simulink model "x2dof_manipulator_sim"  (R2025b)
settings: Solver=ode23t  StartTime=0.0  StopTime=simtime  RelTol=1e-3
values from neighbouring files (symbols this model uses):
  Kd = 3    [manip_parameters.m]
  Kp = 10    [manip_parameters.m]
  l1 = 0.6658    [manip_parameters.m]    (also in simscape_fitness.m = x(1))
  l2 = 0.3342    [manip_parameters.m]    (also in simscape_fitness.m = x(2))
  M = 5    [manip_parameters.m]
  R1 = 0.0102    [manip_parameters.m]    (also in simscape_fitness.m = x(3))
  R2 = 0.0101    [manip_parameters.m]    (also in simscape_fitness.m = x(4))
  thickness = 2/1000    (= 0.002)    [manip_parameters.m]
  X0 = l1    (= 0.6658)    [manip_parameters.m]
  Xf = 0.1    [manip_parameters.m]
  Z0 = (l1^2+l2^2)^(1/2)    (= 0.744969314804)    [manip_parameters.m]
  Zf = 0.5    [manip_parameters.m]
undefined symbols (not defined in the file or in its folder): X, Y, Z
libraries: sm_lib x12, nesl_utility x10
settings Model: Creator=david  LastModifiedBy=david
settings ExplorerConfigSet: InternalSimMechanicsExplorerSettings=|
  | <ExplorerConfiguration>
  | 
  |   <canonicalview>default</canonicalview>
  | 
  |   <TilePanel>
  |     <TileInfo>
  |       <Tiles Columns="1" Count="1" Height="608" Rows="1" Width="1079">
  |         <Row Weight="1"/>
  |         <Column Weight="1"/>
  |         <Tile Height="1" Width="1" X="0" Y="0"/>
  |       </Tiles>
  |     </TileInfo>
  |     <SceneInfo>
  |       <SceneViewer>
  |         <IsThisViewStd>
  |           <IsStandardView>off</IsStandardView>
  |           <StandardViewName>Front</StandardViewName>
  |         </IsThisViewStd>
  |         <BGColor>
  |           <R>1</R>
  |           <G>1</G>
  |           <B>1</B>
  |           <A>1</A>
  |         </BGColor>
  |         <Camera>
  |           <DoPerspective>off</DoPerspective>
  |           <Position>
  |             <X>0.46670638678844834</X>
  |             <Y>-2.3711199999999999</Y>
  |             <Z>0.2607597590218651</Z>
  |           </Position>
  |           <Center>
  |             <X>0.46670638678844834</X>
  |             <Y>0</Y>
  |             <Z>0.2607597590218651</Z>
  |           </Center>
  |           <Up>
  |             <X>0</X>
  |             <Y>0</Y>
  |             <Z>1</Z>
  |           </Up>
  |           <XLim>0.53368918601454662</XLim>
  |           <YLim>0.53368918601454662</YLim>
  |           <ViewLimDist>0.01</ViewLimDist>
  |         </Camera>
  |       </SceneViewer>
  |     </SceneInfo>
  |   </TilePanel>
  | 
  |   <MechEditorPanel>
  |     <GfxPanelCameraMap/>
  |     <Cameras/>
  |     <VideoCreator>
  |       <IncludeTiles>All</IncludeTiles>
  |       <IncludeTime>on</IncludeTime>
  |       <IncludeWorldFrame>off</IncludeWorldFrame>
  |       <PlaybackSpeedRatio>1</PlaybackSpeedRatio>
  |       <FrameRate>30</FrameRate>
  |       <FrameSize>auto</FrameSize>
  |       <VideoFormat>UncompressedAVI</VideoFormat>
  |     </VideoCreator>
  |   </MechEditorPanel>
  | 
  |   <PlaybackSettings>
  |     <PlaybackSpeedFactor>1</PlaybackSpeedFactor>
  |   </PlaybackSettings>
  | 
  | </ExplorerConfiguration>

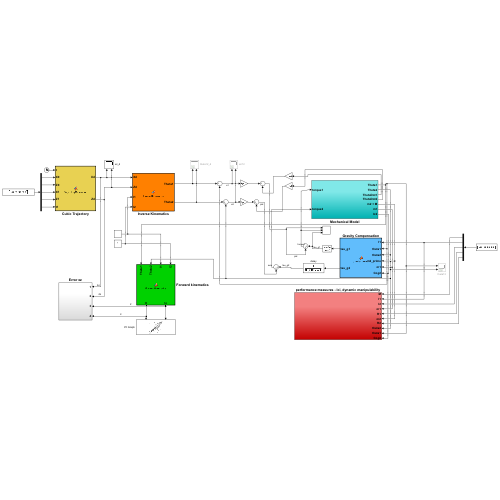
[thumbnail: Simulink's stored preview of the top-level diagram]
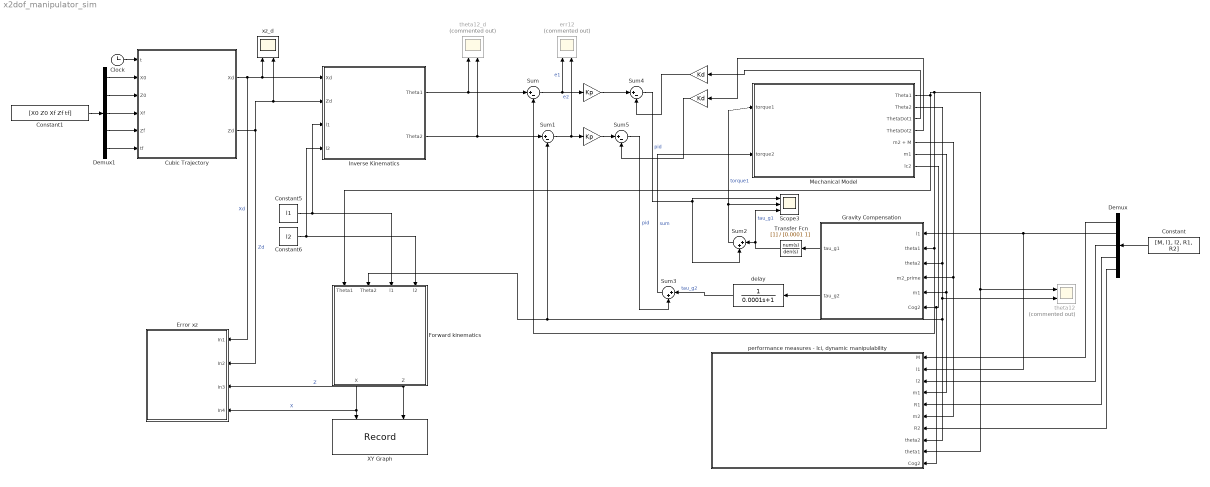
== system x2dof_manipulator_sim ==
  " " : Gain  Gain=Kd
  "  " : Gain  Gain=Kd
  "    " : Gain  Gain=Kp
  "     " : Gain  Gain=Kp
  Clock : Clock
  Constant : Constant  Value=[M, l1, l2, R1, R2]
  Constant1 : Constant  Value=[X0 Z0 Xf Zf tf]
  Constant5 : Constant  Value=l1
  Constant6 : Constant  Value=l2
  Cubic Trajectory : MATLAB Function  TreatAsAtomicUnit=on
  Demux : Demux  Outputs=5
  Demux1 : Demux  Outputs=5
  Error xz : Subsystem
  Forward kinematics : MATLAB Function  TreatAsAtomicUnit=on
  Gravity Compensation : MATLAB Function  TreatAsAtomicUnit=on
  Inverse Kinematics : MATLAB Function  TreatAsAtomicUnit=on
  Mechanical Model : Subsystem
  Scope3 : Scope  NumInputPorts=3
      settings: ActiveDisplayYMinimum=-28.880542715868771  ActiveDisplayYMaximum=52.065399451376422  DataLoggingVariableName=ScopeData8
  Sum{,1,4..5} (4 alike) : Sum  Inputs=|+-
  Sum2 : Sum  Inputs=|++
  Sum3 : Sum  Inputs=|++
  Transfer Fcn : TransferFcn  Denominator=[0.0001 1]
  XY Graph : Record  NumPorts=2.0  FileSettingsInternal="{\"entries\":[{\"content\":{\"excelSettings\":{\"content\":{},\"type\":\"Streamout.ExcelSettings\"},\"parquetSettings\":{\"content\":{},\"type\":\"Streamout.ParquetSettings\"}},\"type\":\"Streamout.FileSettingStorage\",\"uuid\":\"\"}],\"packageUris\":[\"http:\\/\\/schema.mathworks.com\\/mf0\\/streamout_blocks\\/R2020a\"],\"version\":\"1.0\"}"  FrameSettings=[0, 0]  Layout=[1 1]  SignalsInternal="{\"entries\":[{\"content\":{\"signals\":[{\"content\":{\"blockPath\":[],\"dimensions\":[1],\"domain\":\"\",\"lineColor\":\"#a2142f\",\"plots\":[ 1 ],\"port\":1,\"sid\":[\"\"],\"signalID\":1,\"signalName\":\"X\"},\"type\":\"RecordBlkView.Signal\",\"uuid\":\"\"},{\"content\":{\"blockPath\":[],\"dimensions\":[1],\"domain\":\"\",\"lineColor\":\"#139fff\",\"plots\":[ 1 ],\"port\":2,\"sid\":[\"\"],\"signalID\":2,\"signalName\":\"Z\"},\"type\":\"RecordBlkView.Signal\",\"uuid\":\"\"}]},\"type\":\"RecordBlkView.InputSignals\",\"uuid\":\"\"}],\"packageUris\":[\"http:\\/\\/schema.mathworks.com\\/mf0\\/streamout_blocks\\/R2020a\"],\"version\":\"1.0\"}"  VisualizationBindings="{\"xyplotplugin\":{\"info\":[{\"series\":[{\"bindingParametersList\":[{\"parameter\":\"X-Axis\",\"signalID\":1,\"signalName\":\"X\"},{\"parameter\":\"Y-Axis\",\"signalID\":2,\"signalName\":\"Z\"}],\"seriesID\":0}],\"subplotID\":1}]}}"  CompatibilityTag=XY
  delay : TransferFcn  Denominator=[0.0001 1]
  err12 : Scope  Commented=on  NumInputPorts=2
      settings: ActiveDisplayYMinimum=-1.9844586255520857  ActiveDisplayYMaximum=1.5219369913686587  DataLoggingVariableName=ScopeData10
  "performance measures - lci, dynamic manipulability" : Subsystem
  theta12 : Scope  Commented=on  NumInputPorts=2
      settings: ActiveDisplayYMinimum=-1.6633483735090353  ActiveDisplayYMaximum=1.9932120404099871  DataLoggingVariableName=ScopeData11
  theta12_d : Scope  Commented=on  NumInputPorts=2
      settings: ActiveDisplayYMinimum=-0.67216397152782115  ActiveDisplayYMaximum=3.2154225811620383  DataLoggingVariableName=ScopeData12
  xz_d : Scope  NumInputPorts=2
      settings: ActiveDisplayYMinimum=-1  ActiveDisplayYMaximum=1  DataLoggingVariableName=ScopeData13
  wires:
  Mechanical Model/5(m2 + M) -> Gravity Compensation/4(m2_prime), "performance measures - lci, dynamic manipulability"/6(m2)
  Demux/5 -> "performance measures - lci, dynamic manipulability"/7(R2)
  Demux1/3 -> Cubic Trajectory/4(Xf)
  Inverse Kinematics/2(Theta2) -> theta12_d/2, Sum1/1
  Sum4/1 -> Sum2/2, Scope3/1  "pid"
  Demux/1 -> "performance measures - lci, dynamic manipulability"/1(M)
  Sum5/1 -> Sum3/2  "pid"
  Demux1/5 -> Cubic Trajectory/6(tf)
  Constant1/1 -> Demux1/1
  Constant/1 -> Demux/1
  Demux1/2 -> Cubic Trajectory/3(Z0)
  Mechanical Model/1(Theta1) -> Forward kinematics/1(Theta1), Gravity Compensation/2(theta1), Sum/2, theta12/1, "performance measures - lci, dynamic manipulability"/9(theta1)
  "    "/1 -> Sum5/1
  Transfer Fcn/1 -> Scope3/3, Sum2/1  "tau_g1"
  Cubic Trajectory/1(Xd) -> Error xz/1(In1), Inverse Kinematics/1(Xd), xz_d/1  "Xd"
  "  "/1 -> Sum4/2
  Demux/3 -> "performance measures - lci, dynamic manipulability"/3(l2)
  delay/1 -> Sum3/1  "tau_g2"
  Gravity Compensation/2(tau_g2) -> delay/1
  Forward kinematics/2(Z) -> Error xz/3(In3), XY Graph/2  "Z"
  Gravity Compensation/1(tau_g1) -> Transfer Fcn/1
  Demux/4 -> "performance measures - lci, dynamic manipulability"/5(R1)
  Forward kinematics/1(X) -> Error xz/4(In4), XY Graph/1  "X"
  Mechanical Model/6(m1) -> Gravity Compensation/5(m1), "performance measures - lci, dynamic manipulability"/4(m1)
  Demux1/4 -> Cubic Trajectory/5(Zf)
  Sum2/1 -> Scope3/2, Mechanical Model/1(torque1)  "torque1"
  Demux1/1 -> Cubic Trajectory/2(X0)
  Mechanical Model/3(ThetaDot1) -> "  "/1
  Sum3/1 -> Mechanical Model/2(torque2)  "sum"
  Constant5/1 -> Forward kinematics/3(l1), Inverse Kinematics/3(l1)
  Demux/2 -> Gravity Compensation/1(l1), "performance measures - lci, dynamic manipulability"/2(l1)
  "     "/1 -> Sum4/1
  " "/1 -> Sum5/2
  Mechanical Model/2(Theta2) -> theta12/2, Sum1/2, Forward kinematics/2(Theta2), "performance measures - lci, dynamic manipulability"/8(theta2), Gravity Compensation/3(theta2)
  Sum1/1 -> err12/2, "    "/1  "e2"
  Mechanical Model/7(lc2) -> Gravity Compensation/6(Cog2), "performance measures - lci, dynamic manipulability"/10(Cog2)
  Sum/1 -> err12/1, "     "/1  "e1"
  Cubic Trajectory/2(Zd) -> Error xz/2(In2), xz_d/2, Inverse Kinematics/2(Zd)  "Zd"
  Clock/1 -> Cubic Trajectory/1(t)
  Mechanical Model/4(ThetaDot2) -> " "/1
  Inverse Kinematics/1(Theta1) -> theta12_d/1, Sum/1
  Constant6/1 -> Forward kinematics/4(l2), Inverse Kinematics/4(l2)

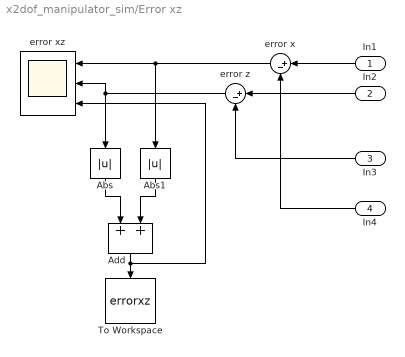
== system x2dof_manipulator_sim/Error xz ==
  In1 : Inport
  In2 : Inport  Port=2
  In3 : Inport  Port=3
  In4 : Inport  Port=4
  Abs : Abs  SaturateOnIntegerOverflow=off
  Abs1 : Abs  SaturateOnIntegerOverflow=off
  Add : Sum
  To Workspace : ToWorkspace  VariableName=errorxz  SampleTime=-1
  error x : Sum  Inputs=|+-
  error xz : Scope  NumInputPorts=3
      settings: ActiveDisplayYMinimum=-1.795161966927977  ActiveDisplayYMaximum=2.51299530874783  DataLoggingVariableName=ScopeData5
  error z : Sum  Inputs=|+-
  wires:
  In3/1 -> error z/2
  In1/1 -> error x/1
  Abs1/1 -> Add/2
  error x/1 -> error xz/1, Abs1/1
  In4/1 -> error x/2
  In2/1 -> error z/1
  Abs/1 -> Add/1
  Add/1 -> To Workspace/1, error xz/3
  error z/1 -> error xz/2, Abs/1

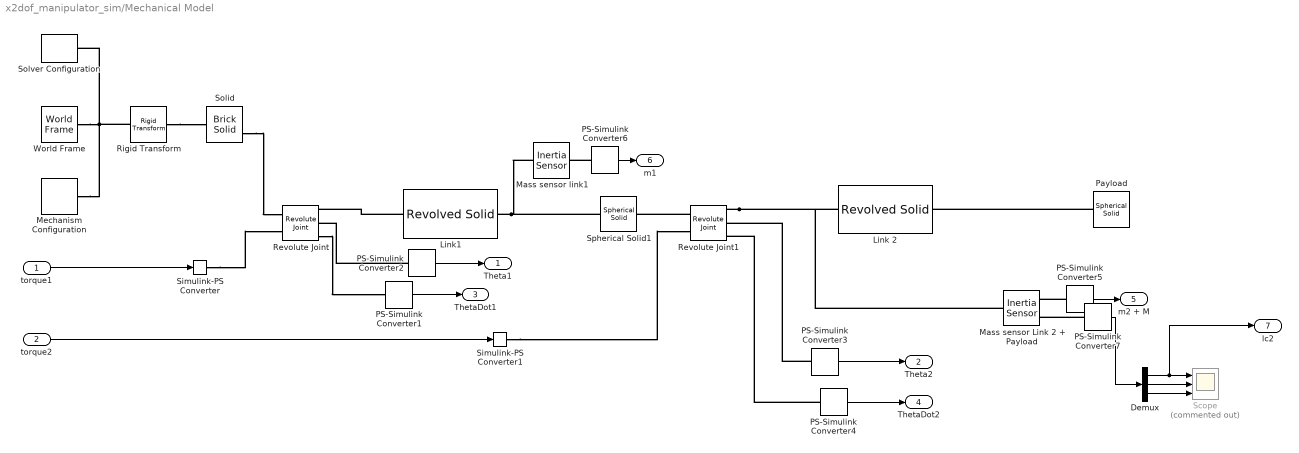
== system x2dof_manipulator_sim/Mechanical Model ==
  torque1 : Inport
  torque2 : Inport  Port=2
  Demux : Demux  Outputs=3
  Link 2 : sm_lib/Body Elements/Revolved Solid  RevolutionCrossSection=[(R2-thickness), -l2/2; R2, -l2/2; R2, l2/2; (R2-thickness), l2/2]  RevolutionCrossSectionUnits=m  RevolutionExtent=Full  RevolutionAngle=180  RevolutionAngleUnits=deg  ExportConvexHullGeometry=off  InertiaType=CalculateFromGeometry  BasedOnType=Density  Density=2640.28  DensityUnits=kg/m^3  Mass=1  MassUnits=kg  CenterOfMass=[0 0 0]  CenterOfMassUnits=m  MomentsOfInertia=[1 1 1]  MomentsOfInertiaUnits=kg*m^2  ProductsOfInertia=[0 0 0]  ProductsOfInertiaUnits=kg*m^2  GraphicType=FromGeometry  MarkerShape=Sphere  MarkerSize=10  GraphicVisPropType=SimpleVisualProperties  GraphicDiffuseColor=[0.5 0.5 0.5]  GraphicOpacity=1  GraphicSpecularColor=[0.5 0.5 0.5 1.0]  GraphicAmbientColor=[0.15 0.15 0.15 1.0]  GraphicEmissiveColor=[0.0 0.0 0.0 1.0]  GraphicShininess=75  DoExposeReferenceFrame=off  SerializedFrames=|
      | <Frames>
      | 
      |   <Frame>
      |     <Id>Frame1</Id>
      |     <Value>
      |       <Name>L</Name>
      |       <Origin>
      |         <Source>GeometricFeature</Source>
      |         <FeatureName>side curve 3</FeatureName>
      |       </Origin>
      |       <PrimaryAxis>
      |         <DefinedDirection>+Z</DefinedDirection>
      |         <Source>ReferenceFrame</Source>
      |         <SourceDirection>-X</SourceDirection>
      |         <FeatureName></FeatureName>
      |       </PrimaryAxis>
      |       <SecondaryAxis>
      |         <DefinedDirection>+Y</DefinedDirection>
      |         <Source>ReferenceFrame</Source>
      |         <SourceDirection>-Y</SourceDirection>
      |         <FeatureName></FeatureName>
      |       </SecondaryAxis>
      |     </Value>
      |   </Frame>
      | 
      |   <Frame>
      |     <Id>Frame2</Id>
      |     <Value>
      |       <Name>R</Name>
      |       <Origin>
      |         <Source>GeometricFeature</Source>
      |         <FeatureName>side surface 1</FeatureName>
      |       </Origin>
      |       <PrimaryAxis>
      |         <DefinedDirection>+Z</DefinedDirection>
      |         <Source>ReferenceFrame</Source>
      |         <SourceDirection>-X</SourceDirection>
      |         <FeatureName></FeatureName>
      |       </PrimaryAxis>
      |       <SecondaryAxis>
      |         <DefinedDirection>+Y</DefinedDirection>
      |         <Source>ReferenceFrame</Source>
      |         <SourceDirection>-Y</SourceDirection>
      |         <FeatureName></FeatureName>
      |       </SecondaryAxis>
      |     </Value>
      |   </Frame>
      | 
      | </Frames>
  "Link1 " : sm_lib/Body Elements/Revolved Solid  RevolutionCrossSection=[(R1-thickness), -l1/2; R1, -l1/2; R1, l1/2; (R1-thickness), l1/2]  RevolutionCrossSectionUnits=m  RevolutionExtent=Full  RevolutionAngle=180  RevolutionAngleUnits=deg  ExportConvexHullGeometry=off  InertiaType=CalculateFromGeometry  BasedOnType=Density  Density=2640.28  DensityUnits=kg/m^3  Mass=1  MassUnits=kg  CenterOfMass=[0 0 0]  CenterOfMassUnits=m  MomentsOfInertia=[1 1 1]  MomentsOfInertiaUnits=kg*m^2  ProductsOfInertia=[0 0 0]  ProductsOfInertiaUnits=kg*m^2  GraphicType=FromGeometry  MarkerShape=Sphere  MarkerSize=10  GraphicVisPropType=SimpleVisualProperties  GraphicDiffuseColor=[0.5 0.5 0.5]  GraphicOpacity=1  GraphicSpecularColor=[0.5 0.5 0.5 1.0]  GraphicAmbientColor=[0.15 0.15 0.15 1.0]  GraphicEmissiveColor=[0.0 0.0 0.0 1.0]  GraphicShininess=75  DoExposeReferenceFrame=off  SerializedFrames=|
      | <Frames>
      | 
      |   <Frame>
      |     <Id>Frame1</Id>
      |     <Value>
      |       <Name>L</Name>
      |       <Origin>
      |         <Source>GeometricFeature</Source>
      |         <FeatureName>side curve 3</FeatureName>
      |       </Origin>
      |       <PrimaryAxis>
      |         <DefinedDirection>+Z</DefinedDirection>
      |         <Source>ReferenceFrame</Source>
      |         <SourceDirection>-X</SourceDirection>
      |         <FeatureName></FeatureName>
      |       </PrimaryAxis>
      |       <SecondaryAxis>
      |         <DefinedDirection>+Y</DefinedDirection>
      |         <Source>ReferenceFrame</Source>
      |         <SourceDirection>-Y</SourceDirection>
      |         <FeatureName></FeatureName>
      |       </SecondaryAxis>
      |     </Value>
      |   </Frame>
      | 
      |   <Frame>
      |     <Id>Frame2</Id>
      |     <Value>
      |       <Name>R</Name>
      |       <Origin>
      |         <Source>GeometricFeature</Source>
      |         <FeatureName>side surface 1</FeatureName>
      |       </Origin>
      |       <PrimaryAxis>
      |         <DefinedDirection>+Z</DefinedDirection>
      |         <Source>ReferenceFrame</Source>
      |         <SourceDirection>-X</SourceDirection>
      |         <FeatureName></FeatureName>
      |       </PrimaryAxis>
      |       <SecondaryAxis>
      |         <DefinedDirection>+Y</DefinedDirection>
      |         <Source>ReferenceFrame</Source>
      |         <SourceDirection>-Y</SourceDirection>
      |         <FeatureName></FeatureName>
      |       </SecondaryAxis>
      |     </Value>
      |   </Frame>
      | 
      | </Frames>
  Mass sensor Link 2 + Payload : sm_lib/Body Elements/Inertia Sensor  SensorExtent=BodyGroup  SpanWeldJoints=off  ExcludeGroundedBodies=off  MeasurementFrame=Attached  SenseMass=on  SenseCenterOfMass=on  SenseInertiaMatrix=off  SenseCenteredInertiaMatrix=off  SensePrincipalInertiaMatrix=off  SenseRotationMatrix=off  GraphicType=PrincipalInertiaFrame  PrincipalInertiaFrameSize=20  GraphicVisPropType=SimpleVisualProperties  GraphicDiffuseColor=[0.5 0.5 0.5]  GraphicOpacity=1  GraphicSpecularColor=[0.5 0.5 0.5 1.0]  GraphicAmbientColor=[0.15 0.15 0.15 1.0]  GraphicEmissiveColor=[0.0 0.0 0.0 1.0]  GraphicShininess=75
  "Mass sensor link1 " : sm_lib/Body Elements/Inertia Sensor  SensorExtent=BodyGroup  SpanWeldJoints=off  ExcludeGroundedBodies=off  MeasurementFrame=Attached  SenseMass=on  SenseCenterOfMass=off  SenseInertiaMatrix=off  SenseCenteredInertiaMatrix=off  SensePrincipalInertiaMatrix=off  SenseRotationMatrix=off  GraphicType=PrincipalInertiaFrame  PrincipalInertiaFrameSize=20  GraphicVisPropType=SimpleVisualProperties  GraphicDiffuseColor=[0.5 0.5 0.5]  GraphicOpacity=1  GraphicSpecularColor=[0.5 0.5 0.5 1.0]  GraphicAmbientColor=[0.15 0.15 0.15 1.0]  GraphicEmissiveColor=[0.0 0.0 0.0 1.0]  GraphicShininess=75
  Mechanism Configuration : sm_lib/Utilities/Mechanism Configuration  UniformGravity=Constant  GravityVector=[0 0 -9.81]  GravityVectorUnits=m/s^2  LinearizationDelta=0.001  JointModeTransitionNonlinearIterations=2
  PS-Simulink Converter{1..6} (6 alike) : nesl_utility/PS-Simulink Converter  PhysicalDomain=network_engine_domain  SubClassName=ps_output  LeftPortType=input  RightPortType=output  PseudoPeriodic=off  Frequencies=[]  VectorFormat=1-D array  Unit=1  AffineConversion=off
  PS-Simulink Converter7 : nesl_utility/PS-Simulink Converter  PhysicalDomain=network_engine_domain  SubClassName=ps_output  LeftPortType=input  RightPortType=output  PseudoPeriodic=off  Frequencies=[]  VectorFormat=1-D array  Unit=m  AffineConversion=off
  Payload : sm_lib/Body Elements/Spherical Solid  SphereRadius=2*R2  SphereRadiusUnits=m  ExportEntireGeometry=off  InertiaType=CalculateFromGeometry  BasedOnType=Mass  Density=1000  DensityUnits=kg/m^3  Mass=M  MassUnits=kg  CenterOfMass=[0 0 0]  CenterOfMassUnits=m  MomentsOfInertia=[1 1 1]  MomentsOfInertiaUnits=kg*m^2  ProductsOfInertia=[0 0 0]  ProductsOfInertiaUnits=kg*m^2  GraphicType=FromGeometry  MarkerShape=Sphere  MarkerSize=10  GraphicVisPropType=SimpleVisualProperties  GraphicDiffuseColor=[0.1529 0.1529 0.1529]  GraphicOpacity=1  GraphicSpecularColor=[0.5 0.5 0.5 1.0]  GraphicAmbientColor=[0.15 0.15 0.15 1.0]  GraphicEmissiveColor=[0.0 0.0 0.0 1.0]  GraphicShininess=75  DoExposeReferenceFrame=on  SerializedFrames=<Frames/>
  Revolute Joint : sm_lib/Joints/Revolute Joint  JointMode=Normal  CompositeWrenchDir=FollowerOnBase  CompositeWrenchFrame=BaseFrame  SenseConstraintForce=off  SenseConstraintTorque=off  SenseTotalForce=off  SenseTotalTorque=off  PositionTargetSpecify=on  PositionTargetPriority=High  PositionTargetValue=0  PositionTargetValueUnits=rad  VelocityTargetSpecify=off  VelocityTargetPriority=High  VelocityTargetValue=0  VelocityTargetValueUnits=deg/s  EquilibriumPosition=0  EquilibriumPositionUnits=rad  SpringStiffness=0  SpringStiffnessUnits=N*m/deg  DampingCoefficient=0  DampingCoefficientUnits=N*m/(deg/s)  LowerLimitSpecify=on  LowerLimitBound=0  LowerLimitBoundUnits=rad  LowerLimitStiffness=1e4  LowerLimitStiffnessUnits=N*m/deg  LowerLimitDamping=10  LowerLimitDampingUnits=N*m/(deg/s)  LowerLimitTransitionRegionWidth=0.1  LowerLimitTransitionRegionWidthUnits=deg  UpperLimitSpecify=on  UpperLimitBound=pi  UpperLimitBoundUnits=rad  UpperLimitStiffness=1e4  UpperLimitStiffnessUnits=N*m/deg  UpperLimitDamping=10  UpperLimitDampingUnits=N*m/(deg/s)  UpperLimitTransitionRegionWidth=0.1  UpperLimitTransitionRegionWidthUnits=deg  TorqueActuationMode=InputTorque  MotionActuationMode=ComputedMotion  SensePosition=on  SenseVelocity=on  SenseAcceleration=off  SenseTorqueForce=off  SenseLowerLimitTorqueForce=off  SenseUpperLimitTorqueForce=off
  Revolute Joint1 : sm_lib/Joints/Revolute Joint  JointMode=Normal  CompositeWrenchDir=BaseOnFollower  CompositeWrenchFrame=BaseFrame  SenseConstraintForce=off  SenseConstraintTorque=off  SenseTotalForce=off  SenseTotalTorque=off  PositionTargetSpecify=on  PositionTargetPriority=High  PositionTargetValue=pi/2  PositionTargetValueUnits=rad  VelocityTargetSpecify=off  VelocityTargetPriority=High  VelocityTargetValue=0  VelocityTargetValueUnits=deg/s  EquilibriumPosition=pi/2  EquilibriumPositionUnits=rad  SpringStiffness=0  SpringStiffnessUnits=N*m/deg  DampingCoefficient=0  DampingCoefficientUnits=N*m/(deg/s)  LowerLimitSpecify=on  LowerLimitBound=-2.9  LowerLimitBoundUnits=rad  LowerLimitStiffness=1e4  LowerLimitStiffnessUnits=N*m/deg  LowerLimitDamping=10  LowerLimitDampingUnits=N*m/(deg/s)  LowerLimitTransitionRegionWidth=0.1  LowerLimitTransitionRegionWidthUnits=deg  UpperLimitSpecify=on  UpperLimitBound=2.9  UpperLimitBoundUnits=rad  UpperLimitStiffness=1e4  UpperLimitStiffnessUnits=N*m/deg  UpperLimitDamping=10  UpperLimitDampingUnits=N*m/(deg/s)  UpperLimitTransitionRegionWidth=0.1  UpperLimitTransitionRegionWidthUnits=deg  TorqueActuationMode=InputTorque  MotionActuationMode=ComputedMotion  SensePosition=on  SenseVelocity=on  SenseAcceleration=off  SenseTorqueForce=off  SenseLowerLimitTorqueForce=off  SenseUpperLimitTorqueForce=off
  Rigid Transform : sm_lib/Frames and Transforms/Rigid Transform  RotationMethod=StandardAxis  FollAlignAxisA=+X  BaseAlignAxisA=+Y  FollAlignAxisB=+Y  BaseAlignAxisB=+Z  RotationStandardAxis=-X  RotationAngle=-90  RotationAngleUnits=deg  RotationArbitraryAxis=[0 0 1]  RotationSequenceAxes=FollowerAxes  RotationSequence=XYX  RotationSequenceAngles=[0 0 0]  RotationSequenceAnglesUnits=deg  RotationMatrix=[1 0 0;0 1 0;0 0 1]  Quaternion=[1 0 0 0]  TranslationMethod=None  TranslationCartesianOffset=[0 0 0]  TranslationCartesianOffsetUnits=m  TranslationStandardAxis=+Z  TranslationStandardOffset=0  TranslationStandardOffsetUnits=m  TranslationROffset=0  TranslationROffsetUnits=m  TranslationThetaOffset=0  TranslationThetaOffsetUnits=deg  TranslationZOffset=0  TranslationZOffsetUnits=m
  Scope : Scope  Commented=on  NumInputPorts=3
      settings: ActiveDisplayYMinimum=0.2660004265435636  ActiveDisplayYMaximum=0.46600042654356366  DataLoggingVariableName=ScopeData9
  Simulink-PS Converter : nesl_utility/Simulink-PS Converter  PhysicalDomain=network_engine_domain  SubClassName=ps_input  LeftPortType=input  RightPortType=output  PseudoPeriodic=off  Frequencies=[]  NoiseDistribution=none  NoiseParameters=[]  Unit=1  AffineConversion=off  FilteringAndDerivatives=provide  SimscapeFilterOrder=1  InputFilterTimeConstant=0.001  UdotUserProvided=0
  Simulink-PS Converter1 : nesl_utility/Simulink-PS Converter  PhysicalDomain=network_engine_domain  SubClassName=ps_input  LeftPortType=input  RightPortType=output  PseudoPeriodic=off  Frequencies=[]  NoiseDistribution=none  NoiseParameters=[]  Unit=1  AffineConversion=off  FilteringAndDerivatives=provide  SimscapeFilterOrder=1  InputFilterTimeConstant=0.001  UdotUserProvided=0
  Solid : sm_lib/Body Elements/Brick Solid  BrickDimensions=[3*R1 R1*3 R1*3]  BrickDimensionsUnits=m  ExportEntireGeometry=off  InertiaType=CalculateFromGeometry  BasedOnType=Mass  Density=2640.28  DensityUnits=kg/m^3  Mass=0  MassUnits=kg  CenterOfMass=[0 0 0]  CenterOfMassUnits=m  MomentsOfInertia=[1 1 1]  MomentsOfInertiaUnits=kg*m^2  ProductsOfInertia=[1 1 1]  ProductsOfInertiaUnits=kg*m^2  GraphicType=FromGeometry  MarkerShape=Sphere  MarkerSize=10  GraphicVisPropType=SimpleVisualProperties  GraphicDiffuseColor=[0.0 0.0 0.6]  GraphicOpacity=1.0  GraphicSpecularColor=[0.5 0.5 0.5 1.0]  GraphicAmbientColor=[0.15 0.15 0.15 1.0]  GraphicEmissiveColor=[0.0 0.0 0.0 1.0]  GraphicShininess=75  DoExposeReferenceFrame=on  SerializedFrames=|
      | <Frames>
      | 
      |   <Frame>
      |     <Id>Frame1</Id>
      |     <Value>
      |       <Name>F</Name>
      |       <Origin>
      |         <Source>GeometricFeature</Source>
      |         <FeatureName>-z surface</FeatureName>
      |       </Origin>
      |       <PrimaryAxis>
      |         <DefinedDirection>+Z</DefinedDirection>
      |         <Source>ReferenceFrame</Source>
      |         <SourceDirection>+Z</SourceDirection>
      |         <FeatureName></FeatureName>
      |       </PrimaryAxis>
      |       <SecondaryAxis>
      |         <DefinedDirection>+X</DefinedDirection>
      |         <Source>ReferenceFrame</Source>
      |         <SourceDirection>+X</SourceDirection>
      |         <FeatureName></FeatureName>
      |       </SecondaryAxis>
      |     </Value>
      |   </Frame>
      | 
      |   <Frame>
      |     <Id>Frame2</Id>
      |     <Value>
      |       <Name>F2</Name>
      |       <Origin>
      |         <Source>ReferenceFrame</Source>
      |         <FeatureName></FeatureName>
      |       </Origin>
      |       <PrimaryAxis>
      |         <DefinedDirection>+Z</DefinedDirection>
      |         <Source>ReferenceFrame</Source>
      |         <SourceDirection>+Z</SourceDirection>
      |         <FeatureName></FeatureName>
      |       </PrimaryAxis>
      |       <SecondaryAxis>
      |         <DefinedDirection>+X</DefinedDirection>
      |         <Source>ReferenceFrame</Source>
      |         <SourceDirection>+X</SourceDirection>
      |         <FeatureName></FeatureName>
      |       </SecondaryAxis>
      |     </Value>
      |   </Frame>
      | 
      | </Frames>
  Solver Configuration : nesl_utility/Solver Configuration  PhysicalDomain=network_engine_domain  SubClassName=solver  LeftPortType=input  RightPortType=generic  Tones=[]  Harmonics=[]  SimulateNoise=off  Profile=off  UseLocalSampling=off  EnableSwitchedLinearOptims=on  FrequencyDomain=off  UseCCode=off  RelTol=0.001  AbsTol=1e-06  MinStep=1e-09  ToWorkspace=off  RevertToSquareIcSolve=off  NumHomotopyIterations=100  PhasorMode=off  PhasorModeNumHarmonics=1  ConsistencySolver=NEWTON_FTOL  IndexReductionMethod=DerivativeReplacement  DoDC=off  ResidualTolerance=1e-09  ConsistencyTolSource=GLOBAL  ConsistencyAbsTol=0.001  ConsistencyRelTol=0.001  ConsistencyTolFactor=0.001  UseLocalSolver=off  LocalSolverChoice=NE_BACKWARD_EULER_ADVANCER  ResolveIndetEquations=on  FunctionEvalNumThread=1  LocalSolverSampleTime=0.001  DoFixedCost=off  MaxNonlinIter=3  MaxModeIter=2  ComputeImpulses=off  ImpulseIterations=2  LinearAlgebra=Sparse  LinearAlgebraNumThread=0  EquationFormulation=NE_TIME_EF  DelaysMemoryBudget=1024  AutomaticFiltering=on  FilteringTimeConstant=0.001  PartitionStorageMethod=AS_NEEDED  PartitionMemoryBudget=1024  PartitionMethod=FAST  MultibodyUseLocalSolver=off  MultibodyLocalSolverChoice=ODE1  MultibodyLocalSolverSampleTime=0.001
  Spherical Solid1 : sm_lib/Body Elements/Spherical Solid  SphereRadius=R1  SphereRadiusUnits=m  ExportEntireGeometry=off  InertiaType=CalculateFromGeometry  BasedOnType=Mass  Density=1000  DensityUnits=kg/m^3  Mass=0  MassUnits=kg  CenterOfMass=[0 0 0]  CenterOfMassUnits=m  MomentsOfInertia=[1 1 1]  MomentsOfInertiaUnits=kg*m^2  ProductsOfInertia=[0 0 0]  ProductsOfInertiaUnits=kg*m^2  GraphicType=FromGeometry  MarkerShape=Sphere  MarkerSize=10  GraphicVisPropType=SimpleVisualProperties  GraphicDiffuseColor=[0 0 0]  GraphicOpacity=1  GraphicSpecularColor=[0.5 0.5 0.5 1.0]  GraphicAmbientColor=[0.15 0.15 0.15 1.0]  GraphicEmissiveColor=[0.0 0.0 0.0 1.0]  GraphicShininess=75  DoExposeReferenceFrame=on  SerializedFrames=|
      | <Frames>
      | 
      |   <Frame>
      |     <Id>Frame1</Id>
      |     <Value>
      |       <Name>R2</Name>
      |       <Origin>
      |         <Source>ReferenceFrame</Source>
      |         <FeatureName></FeatureName>
      |       </Origin>
      |       <PrimaryAxis>
      |         <DefinedDirection>+Z</DefinedDirection>
      |         <Source>ReferenceFrame</Source>
      |         <SourceDirection>+Z</SourceDirection>
      |         <FeatureName></FeatureName>
      |       </PrimaryAxis>
      |       <SecondaryAxis>
      |         <DefinedDirection>+X</DefinedDirection>
      |         <Source>ReferenceFrame</Source>
      |         <SourceDirection>+X</SourceDirection>
      |         <FeatureName></FeatureName>
      |       </SecondaryAxis>
      |     </Value>
      |   </Frame>
      | 
      | </Frames>
  World Frame : sm_lib/Frames and Transforms/World Frame
  Theta1 : Outport  VectorParamsAs1DForOutWhenUnconnected=off
  Theta2 : Outport  Port=2  VectorParamsAs1DForOutWhenUnconnected=off
  ThetaDot1 : Outport  Port=3  VectorParamsAs1DForOutWhenUnconnected=off
  ThetaDot2 : Outport  Port=4  VectorParamsAs1DForOutWhenUnconnected=off
  m2 + M : Outport  Port=5
  m1 : Outport  Port=6
  lc2 : Outport  Port=7
  wires:
  Demux/3 -> Scope/3
  Demux/2 -> Scope/2
  Demux/1 -> lc2/1, Scope/1
  PS-Simulink Converter7/1 -> Demux/1
  PS-Simulink Converter6/1 -> m1/1
  PS-Simulink Converter5/1 -> m2 + M/1
  PS-Simulink Converter4/1 -> ThetaDot2/1
  PS-Simulink Converter1/1 -> ThetaDot1/1
  torque2/1 -> Simulink-PS Converter1/1
  torque1/1 -> Simulink-PS Converter/1
  PS-Simulink Converter3/1 -> Theta2/1
  PS-Simulink Converter2/1 -> Theta1/1
  connections:
  PS-Simulink Converter7/LConn1 -- Mass sensor Link 2 + Payload/RConn2
  PS-Simulink Converter6/LConn1 -- "Mass sensor link1 "/RConn1
  PS-Simulink Converter5/LConn1 -- Mass sensor Link 2 + Payload/RConn1
  "Link1 "/RConn1 -- "Mass sensor link1 "/LConn1 -- Spherical Solid1/RConn1
  PS-Simulink Converter4/LConn1 -- Revolute Joint1/RConn3
  Revolute Joint/RConn3 -- PS-Simulink Converter1/LConn1
  Simulink-PS Converter1/RConn1 -- Revolute Joint1/LConn2
  Simulink-PS Converter/RConn1 -- Revolute Joint/LConn2
  Rigid Transform/RConn1 -- Solid/RConn1
  Payload/RConn1 -- Link 2/RConn1
  "Link1 "/LConn1 -- Revolute Joint/RConn1
  Solid/LConn2 -- Revolute Joint/LConn1
  PS-Simulink Converter2/LConn1 -- Revolute Joint/RConn2
  World Frame/RConn1 -- Rigid Transform/LConn1 -- Mechanism Configuration/RConn1 -- Solver Configuration/RConn1
  PS-Simulink Converter3/LConn1 -- Revolute Joint1/RConn2
  Revolute Joint1/LConn1 -- Spherical Solid1/LConn1
  Revolute Joint1/RConn1 -- Mass sensor Link 2 + Payload/LConn1 -- Link 2/LConn1

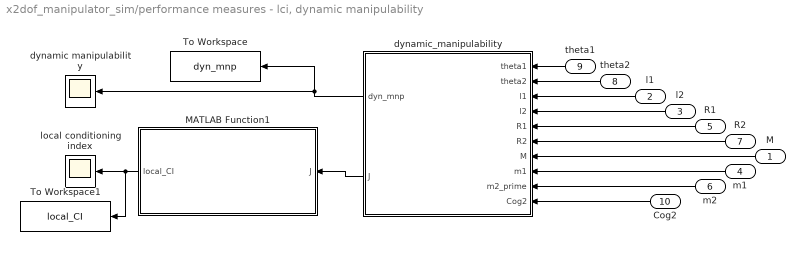
== system x2dof_manipulator_sim/performance measures - lci, dynamic manipulability ==
  M : Inport
  l1 : Inport  Port=2
  l2 : Inport  Port=3
  m1 : Inport  Port=4
  R1 : Inport  Port=5
  m2 : Inport  Port=6
  R2 : Inport  Port=7
  theta2 : Inport  Port=8
  theta1 : Inport  Port=9
  Cog2 : Inport  Port=10
  MATLAB Function1 : MATLAB Function  TreatAsAtomicUnit=on
  To Workspace : ToWorkspace  VariableName=dyn_mnp  SampleTime=-1
  To Workspace1 : ToWorkspace  VariableName=local_CI  SampleTime=-1
  dynamic manipulability : Scope
      settings: ActiveDisplayYMinimum=0.15458196851841136  ActiveDisplayYMaximum=0.34603749870934514  DataLoggingVariableName=ScopeData2
  dynamic_manipulability : MATLAB Function  TreatAsAtomicUnit=on
  local conditioning index : Scope
      settings: ActiveDisplayYMinimum=-0.051608221973677093  ActiveDisplayYMaximum=1.1781205662449763  DataLoggingVariableName=ScopeData7
  wires:
  Cog2/1 -> dynamic_manipulability/10(Cog2)
  l2/1 -> dynamic_manipulability/4(l2)
  M/1 -> dynamic_manipulability/7(M)
  R1/1 -> dynamic_manipulability/5(R1)
  l1/1 -> dynamic_manipulability/3(l1)
  m1/1 -> dynamic_manipulability/8(m1)
  MATLAB Function1/1(local_CI) -> local conditioning index/1, To Workspace1/1
  dynamic_manipulability/2(J) -> MATLAB Function1/1(J)
  theta1/1 -> dynamic_manipulability/1(theta1)
  m2/1 -> dynamic_manipulability/9(m2_prime)
  theta2/1 -> dynamic_manipulability/2(theta2)
  dynamic_manipulability/1(dyn_mnp) -> dynamic manipulability/1, To Workspace/1
  R2/1 -> dynamic_manipulability/6(R2)

== matlab function x2dof_manipulator_sim/Cubic Trajectory ==
  data: t input; Xd output; X0 input; Z0 input; Xf input; Zf input; tf input; Zd output
function [Xd, Zd] = TrajectoryGenerator(t, X0, Z0, Xf, Zf, tf)

% Cubic trajectory setup
% t: current simulation time
% X0, Z0: initial conditions
% Xf, Zf: goal point
% tf: desired time for the total trajectory

    % Keep the time constant so the robot will be still after tf
    if t >= tf
        t = tf;
    end
    
    % time normalization [0-1] for a generalization of the motion law
    tau = t / tf;
    
    % Cubic Polynomial law with initial and final velocity to zero
    s = 3*tau^2 - 2*tau^3;
    
    
    Xd = X0 + (Xf - X0) * s;
    Zd = Z0 + (Zf - Z0) * s;

end

== matlab function x2dof_manipulator_sim/Forward kinematics ==
  data: Theta1 input; X output; Theta2 input; Z output; l1 input; l2 input
function [X,Z] = Forwardkinematics(Theta1, Theta2, l1, l2)

% Forward kinematics based on geometric costruction, xz plane

X=l1*cos(Theta1)+l2*cos(Theta2+Theta1);
Z=l1*sin(Theta1)+l2*sin(Theta2+Theta1);

end

== matlab function x2dof_manipulator_sim/Gravity Compensation ==
  data: l1 input; theta1 input; theta2 input; m2_prime input; tau_g1 output; tau_g2 output; m1 input; Cog2 input
function [tau_g1, tau_g2] = gravity_comp( l1, theta1, theta2, m2_prime, m1, Cog2)
    
    m_motore2 = 0;

    lc1 = l1/2; % CoG link 1 (m)
    lc2 = abs(Cog2); % CoG link 2 (m)
    g = 9.81; % gravity
    
    
    tau_g1 = (m1*lc1 + m_motore2*l1 + (m2_prime)*l1)*g*cos(theta1) + (m2_prime)*lc2*g*cos(theta1 + theta2);
    tau_g2 = (m2_prime)*lc2*g*cos(theta1 + theta2);
    
end

== matlab function x2dof_manipulator_sim/Inverse Kinematics ==
  data: Xd input; Theta1 output; Zd input; Theta2 output; l1 input; l2 input
function [Theta1, Theta2] = InverseKinematics(Xd, Zd, l1, l2)

% The formula derives from the cosine theorem applied to the triangle formed 
% by the two segments of the arm (l1 and l2) and 
% the distance from the origin to the target point.

cos_theta2 = (Xd^2 + Zd^2 - l1^2 - l2^2) / (2 * l1 * l2);

cos_theta2 = max(min(cos_theta2, 1), -1); 

Theta2 = acos(cos_theta2);

s_Theta2 = sin(Theta2);
c_Theta2 = cos(Theta2);

Theta1 = atan2(Zd, Xd) - atan2(l2 * s_Theta2, l1 + l2 * c_Theta2);

end

== matlab function x2dof_manipulator_sim/performance measures - lci, dynamic manipulability/MATLAB Function1 ==
  data: local_CI output; J input
function local_CI = LocalConditioningIndex(J)
    
    s = svd(J);
    
    
    if min(s) < 1e-6
        local_CI = 0; % sigularity case
    else
        k = max(s) / min(s);
        local_CI = 1/k; 
    end
end

== matlab function x2dof_manipulator_sim/performance measures - lci, dynamic manipulability/dynamic_manipulability ==
  data: theta1 input; dyn_mnp output; theta2 input; l1 input; l2 input; R1 input; R2 input; M input; m1 input; m2_prime input; Cog2 input; J output
function [dyn_mnp, J] = dynamic_manipulability(theta1, theta2, l1, l2, R1, R2, M, m1, m2_prime, Cog2)
    
    thickness = 0.002; 
    
    % Internal radii
    r1_in = R1 - thickness;
    r2_in = R2 - thickness;
   
   
    % I = (m/12) * [3*(R_est^2 + R_int^2) + L^2]
    I1 = (m1 / 12) * (3*(R1^2 + r1_in^2) + l1^2);
    I2 = ((m2_prime - M) / 12) * (3*(R2^2 + r2_in^2) + l2^2);
    
    % CoG
    lc1 = l1 / 2;
    lc2 = abs(Cog2);
    
    % For a better representation can be added the motor in the joint, in
    % this case it's not consider
    m_motore2 = 0.0; 
    I_motore = 0;
    
    
    % Jacobian J
    J11 = -l1*sin(theta1) - l2*sin(theta1 + theta2);
    J12 = -l2*sin(theta1 + theta2);
    J21 =  l1*cos(theta1) + l2*cos(theta1 + theta2);
    J22 =  l2*cos(theta1 + theta2);
    
    J = [J11, J12; J21, J22];

    % Mass matrix
    
    M11 = m1*lc1^2 + m_motore2*l1^2 + m2_prime*(l1^2 + lc2^2 + 2*l1*lc2*cos(theta2)) + I1 + I2 + I_motore;
    M12 = m2_prime*(lc2^2 + l1*lc2*cos(theta2)) + I2;
    M21 = M12; 
    M22 = m2_prime*lc2^2 + I2;
    
    
    det_J = J11*J22 - J12*J21; 
    det_M = M11*M22 - M12*M21; 

    % Dynamic manipulability
    
    dyn_mnp = abs(det_J) / det_M;

end
